simulink model "ex01_model"  (R2023a)
settings: Solver=FixedStepDiscrete  StartTime=0.0  StopTime=500*Ts  RelTol=1e-3
values from neighbouring files (symbols this model uses):
  Fc = Fs/16    (= 62500)    [ex00.m]    (also in ex01_config.m; ex02.m = 31250)
  Ts = 1/Fs    (= 1e-06)    [ex01_config.m]    (also in ex02.m; ex03_data.mat)
  x = sin(2*pi*(Fc/Fs)*n)    [ex00.m]    (also in ex01_config.m = flip(x); ex03_data.mat = [0.456261526974 0.188442677697 0.121514194537 0.287000812109)
libraries: dspsrcs4 x2
settings Model: Creator=daniele  LastModifiedBy=mluser
settings SolverCC: AlgebraicLoopSolver=TrustRegion
settings DebuggingCC: UnconnectedInputMsg=warning  UnconnectedOutputMsg=warning  UnconnectedLineMsg=warning
settings ModelReferenceCC: EnableRefExpFcnMdlSchedulingChecks=on
settings RTWCC: DLArmComputeVersion=19.05

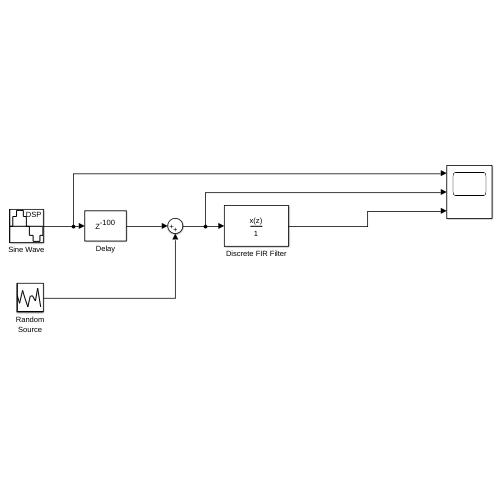
[thumbnail: Simulink's stored preview of the top-level diagram]
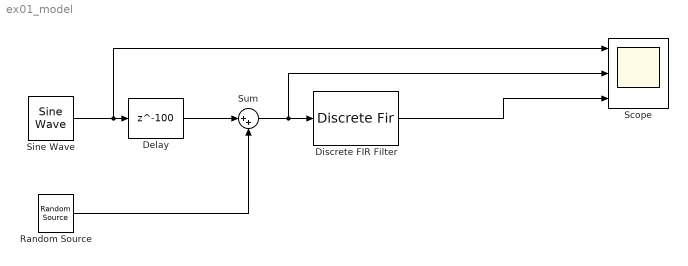
== system ex01_model ==
  Delay : Delay  DelayLength=100  InitialCondition=0
  Discrete FIR Filter : DiscreteFir  Coefficients=x
  Random Source : dspsrcs4/Random Source  SrcType=Gaussian  NormMethod=Ziggurat  CltLength=12  MinVal=0  MaxVal=1  MeanVal=0  VarVal=0.5  RepMode=Not repeatable  rawSeed=1  IsInherit=off  SampMode=Discrete  SampTime=Ts  SampFrame=1  DataType=Double  OutComplex=Real  OutputFrames=off
  Scope : Scope  NumInputPorts=3
  Sine Wave : dspsrcs4/Sine Wave  Amplitude=1  Frequency=Fc  Phase=0  SampleMode=Discrete  OutComplex=Real  CompMethod=Trigonometric fcn  TableSize=Speed  SampleTime=Ts  SamplesPerFrame=1  ResetState=Restart at time zero  OutputFrames=off  dataType=double  wordLen=16  udDataType=sfix(16)  fracBitsMode=Best precision  numFracBits=15  OutDataTypeStr=double  LastOutDataTypeStr=double
  Sum : Sum  Inputs=|++
  wires:
  Sine Wave/1 -> Scope/1, Delay/1
  Delay/1 -> Sum/1
  Random Source/1 -> Sum/2
  Sum/1 -> Scope/2, Discrete FIR Filter/1
  Discrete FIR Filter/1 -> Scope/3
